simulink model "GPS"  (R2023a)
settings: Solver=ode4  StartTime=0.0  StopTime=10.0  FixedStep=dt  RelTol=1e-3
settings Model: Creator=hugobuurmeijer  LastModifiedBy=ndelurgio

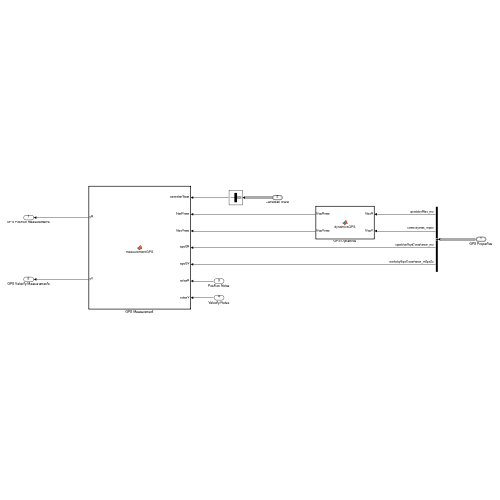
[thumbnail: Simulink's stored preview of the top-level diagram]
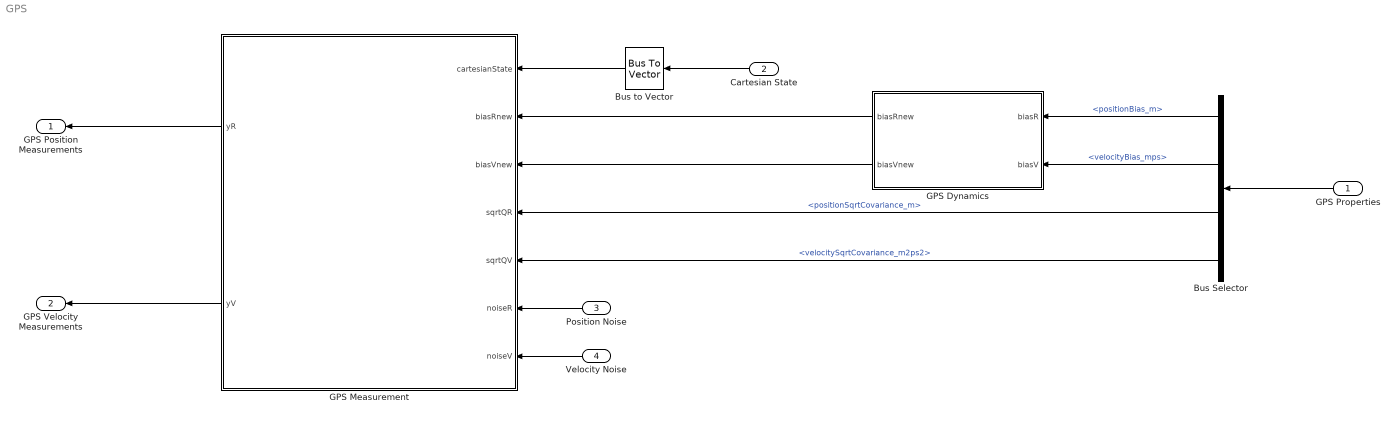
== system GPS ==
  GPS Properties : Inport  OutDataTypeStr=Bus: gps
  Cartesian State : Inport  Port=2  OutDataTypeStr=Bus: cartesianState
  Position Noise : Inport  Port=3  PortDimensions=3
  Velocity Noise : Inport  Port=4  PortDimensions=3
  Bus Selector : BusSelector  OutputSignals=positionBias_m,velocityBias_mps,positionSqrtCovariance_m,velocitySqrtCovariance_m2ps2
  Bus to Vector : BusToVector
  GPS Dynamics : MATLAB Function  TreatAsAtomicUnit=on
  GPS Measurement : MATLAB Function  TreatAsAtomicUnit=on
  GPS Position Measurements : Outport
  GPS Velocity Measurements : Outport  Port=2
  wires:
  GPS Properties/1 -> Bus Selector/1
  Bus Selector/1 -> GPS Dynamics/1(biasR)  "<positionBias_m>"
  GPS Dynamics/1(biasRnew) -> GPS Measurement/2(biasRnew)
  GPS Dynamics/2(biasVnew) -> GPS Measurement/3(biasVnew)
  GPS Measurement/1(yR) -> GPS Position Measurements/1
  GPS Measurement/2(yV) -> GPS Velocity Measurements/1
  Bus Selector/4 -> GPS Measurement/5(sqrtQV)  "<velocitySqrtCovariance_m2ps2>"
  Cartesian State/1 -> Bus to Vector/1
  Bus Selector/2 -> GPS Dynamics/2(biasV)  "<velocityBias_mps>"
  Bus Selector/3 -> GPS Measurement/4(sqrtQR)  "<positionSqrtCovariance_m>"
  Bus to Vector/1 -> GPS Measurement/1(cartesianState)
  Position Noise/1 -> GPS Measurement/6(noiseR)
  Velocity Noise/1 -> GPS Measurement/7(noiseV)

== matlab function GPS/GPS Measurement ==
  data: cartesianState input; yR output; biasRnew input; biasVnew input; sqrtQR input; sqrtQV input; yV output; noiseR input; noiseV input
function [yR, yV] = measurementGPS(cartesianState, biasRnew, biasVnew, sqrtQR, sqrtQV, noiseR, noiseV)

[yR, yV] = measurementGPS(cartesianState, biasRnew, biasVnew, sqrtQR, sqrtQV, noiseR, noiseV);

end

== matlab function GPS/GPS Dynamics ==
  data: biasR input; biasRnew output; biasV input; biasVnew output
function [biasRnew, biasVnew] = dynamicsGPS(biasR, biasV)

[biasRnew, biasVnew] = dynamicsGPS(biasR, biasV);

end
